simulink model "Rotor_old"  (R2018b)
settings: Solver=VariableStepAuto  StartTime=0.0  StopTime=10.0  RelTol=1e-3
settings Model: Creator=Bob  LastModifiedBy=meagh
settings DataIOCC: ReturnWorkspaceOutputs=on
settings RTWCC: Description=FMU Model Exchange 1.0  SystemTargetFile=fmu_me1.tlc  MakeCommand=make_rtw FMIT_INTERMEDIATE_LIB_DIR=DEFAULT  TemplateMakefile=fmu_me1_default_tmf
settings STFCustomTargetCC: TargetLangStandard=C99 (ISO)  ModelReferenceCompliant=off  MATLABClassNameForMDSCustomization=Simulink.SoftwareTarget.TargetSpecificTriggerConfigurationBase  GRTInterface=on  SystemTargetFile=fmu_me1.tlc

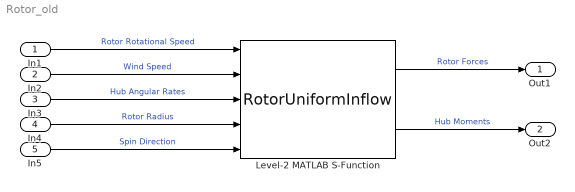
== system Rotor_old ==
  In1 : Inport  OutDataTypeStr=double
  In2 : Inport  Port=2  OutDataTypeStr=double
  In3 : Inport  Port=3  OutDataTypeStr=double
  In4 : Inport  Port=4  OutDataTypeStr=double
  In5 : Inport  Port=5  OutDataTypeStr=boolean
  Level-2 MATLAB S-Function : M-S-Function  FunctionName=RotorUniformInflow
  Out1 : Outport  OutDataTypeStr=double  VectorParamsAs1DForOutWhenUnconnected=off
  Out2 : Outport  Port=2  OutDataTypeStr=double  VectorParamsAs1DForOutWhenUnconnected=off
  wires:
  Level-2 MATLAB S-Function/1 -> Out1/1  "Rotor Forces"
  Level-2 MATLAB S-Function/2 -> Out2/1  "Hub Moments"
  In4/1 -> Level-2 MATLAB S-Function/4  "Rotor Radius"
  In2/1 -> Level-2 MATLAB S-Function/2  "Wind Speed"
  In1/1 -> Level-2 MATLAB S-Function/1  "Rotor Rotational Speed"
  In5/1 -> Level-2 MATLAB S-Function/5  "Spin Direction"
  In3/1 -> Level-2 MATLAB S-Function/3  "Hub Angular Rates"
